simulink model "Indirectimpedance"  (R2017a)
settings: Solver=VariableStepAuto  StartTime=0.0  StopTime=10  RelTol=1e-3
settings Model: Creator=15494  LastModifiedBy=15494

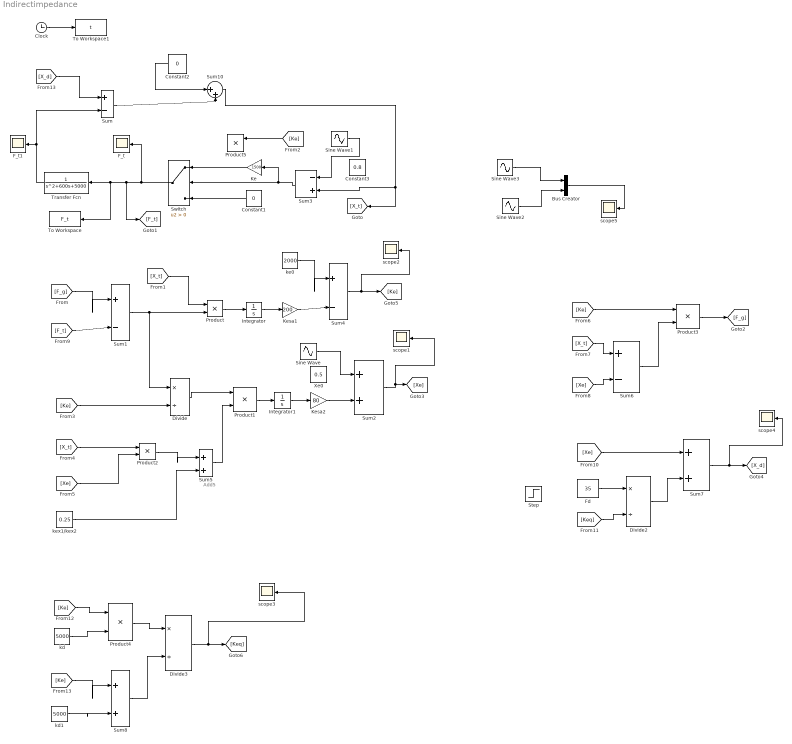
== system Indirectimpedance ==
  note: Add5
  Bus Creator : BusCreator  Inputs=2
  Clock : Clock
  Constant1 : Constant  Value=0
  Constant2 : Constant  Value=0
  Constant3 : Constant  Value=0.8
  Divide : Product  Inputs=*/
  Divide2 : Product  Inputs=*/
  Divide3 : Product  Inputs=*/
  F_t : Scope
  F_t1 : Scope
  Fd : Constant  Value=35
  Integrator : Integrator
  Integrator1 : Integrator
  Ke : Gain  Gain=1500
  Kesa1 : Gain  Gain=200
  Kesa2 : Gain  Gain=80
  Product{,1..5} (6 alike) : Product
  Sine Wave : Sin  Amplitude=0.5  SampleTime=0
  Sine Wave1 : Sin  Amplitude=0.5  Bias=0.2  Phase=0.1  SampleTime=0
  Sine Wave2 : Sin  Amplitude=0.5  SampleTime=0
  Sine Wave3 : Sin  Amplitude=0.5  Bias=0.2  SampleTime=0
  Step : Step  Time=3  Before=50  After=70  SampleTime=0
  Sum : Sum  Inputs=+-
  Sum1 : Sum  Inputs=|+-
  Sum10 : Sum  Inputs=|++
  Sum2 : Sum
  Sum3 : Sum  Inputs=-+
  Sum4 : Sum  Inputs=|+-
  Sum5 : Sum  Inputs=|++
  Sum6 : Sum  Inputs=+-
  Sum7 : Sum
  Sum8 : Sum  Inputs=|++
  Switch : Switch  Criteria=u2 > Threshold
  To Workspace : ToWorkspace  VariableName=F_t  SaveFormat=Timeseries  SampleTime=-1
  To Workspace1 : ToWorkspace  VariableName=t  SaveFormat=Timeseries  SampleTime=-1
  Transfer Fcn : TransferFcn  Denominator=[1 600 5000]
  Xe0 : Constant  Value=0.5
  kd : Constant  Value=5000
  kd1 : Constant  Value=5000
  ke0 : Constant  Value=2000
  kex1/kex2 : Constant  Value=0.25
  scope{1..5} (5 alike) : Scope
  wires:
  Switch/1 -> F_t/1, [F_t], To Workspace/1, Transfer Fcn/1
  Sum3/1 -> Ke/1, Switch/2
  Transfer Fcn/1 -> F_t1/1, Sum/2
  [X_d] -> Sum/1
  Clock/1 -> To Workspace1/1
  [F_g] -> Sum1/1
  [F_t] -> Sum1/2
  Sum1/1 -> Divide/1, Product/2
  [X_t] -> Product/1
  Product/1 -> Integrator/1
  Integrator/1 -> Kesa1/1
  Kesa1/1 -> Sum4/2
  ke0/1 -> Sum4/1
  Sum4/1 -> scope2/1, [Ke]
  [Ke] -> Divide/2
  Divide/1 -> Product1/1
  Product1/1 -> Integrator1/1
  Kesa2/1 -> Sum2/2
  Integrator1/1 -> Kesa2/1
  Sum2/1 -> scope1/1, [Xe]
  [X_t] -> Product2/1
  [Xe] -> Product2/2
  Sum5/1 -> Product1/2
  kex1/kex2/1 -> Sum5/2
  Product2/1 -> Sum5/1
  [Ke] -> Product3/1
  [X_t] -> Sum6/1
  [Xe] -> Sum6/2
  Sum6/1 -> Product3/2
  Product3/1 -> [F_g]
  [Xe] -> Sum7/1
  Divide2/1 -> Sum7/2
  Sum7/1 -> scope4/1, [X_d]
  [Ke] -> Product4/1
  kd/1 -> Product4/2
  Product4/1 -> Divide3/1
  [Ke] -> Sum8/1
  kd1/1 -> Sum8/2
  Sum8/1 -> Divide3/2
  Divide3/1 -> scope3/1, [Keq]
  [Keq] -> Divide2/2
  Sum/1 -> Sum10/2
  Constant2/1 -> Sum10/1
  Sum10/1 -> Sum3/2, [X_t]
  Constant1/1 -> Switch/3
  [Ke] -> Product5/1
  Fd/1 -> Divide2/1
  Ke/1 -> Switch/1
  Sine Wave1/1 -> Sum3/1
  Sine Wave/1 -> Sum2/1
  Sine Wave3/1 -> Bus Creator/1
  Sine Wave2/1 -> Bus Creator/2
  Bus Creator/1 -> scope5/1
